simulink model "Robot_Control"  (R2023b)
settings: Solver=FixedStepDiscrete  StartTime=0.0  StopTime=inf  FixedStep=t_sample  RelTol=1e-3
undefined symbols (not defined in the file): t_sample
settings Model: Creator=FIRSTMentor  LastModifiedBy=ander
settings OptimizationCC: DefaultParameterBehavior=Inlined  StrengthReduction=on  PassReuseOutputArgsAs=Individual arguments  ZeroExternalMemoryAtStartup=off  ZeroInternalMemoryAtStartup=off  OptimizeBlockOrder=speed  OptimizationPriority=Speed  OptimizationCustomize=off  MultiThreadedLoops=on  EfficientTunableParamExpr=on
settings DebuggingCC: MergeDetectMultiDrivingBlocksExec=none  ParameterTunabilityLossMsg=error
settings HardwareCC: ProdBitPerPointer=32  ProdBitPerSizeT=32  ProdBitPerPtrDiffT=32  ProdLargestAtomicInteger=Long  ProdWordSize=32  ProdHWDeviceType=ARM Compatible->ARM 7
settings ModelReferenceCC: PropagateSignalLabelsOutOfModel=off
settings SFSimCC: MATLABDynamicMemAlloc=off
settings RTWCC: Description=Embedded Coder  SystemTargetFile=ert.tlc  GenCodeOnly=on  TemplateMakefile=ert_default_tmf  Toolchain=MinGW64 | gmake (64-bit Windows)
settings CodeAppCC: ForceParamTrailComments=on  IgnoreCustomStorageClasses=off  OperatorAnnotations=on  SimulinkDataObjDesc=on  SFDataObjDesc=on  InsertBlockDesc=on
settings ERTTargetCC: TargetLangStandard=C99 (ISO)  UtilityFuncGeneration=Shared location  SupportVariableSizeSignals=on  ParenthesesLevel=Maximum  InlinedParameterPlacement=NonHierarchical  ERTCustomFileTemplate=example_file_process.tlc

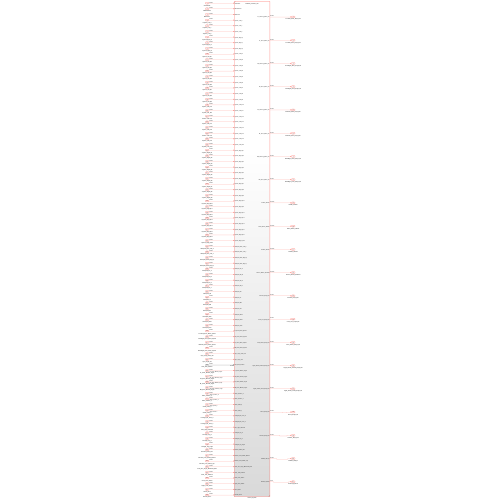
[thumbnail: Simulink's stored preview of the top-level diagram]
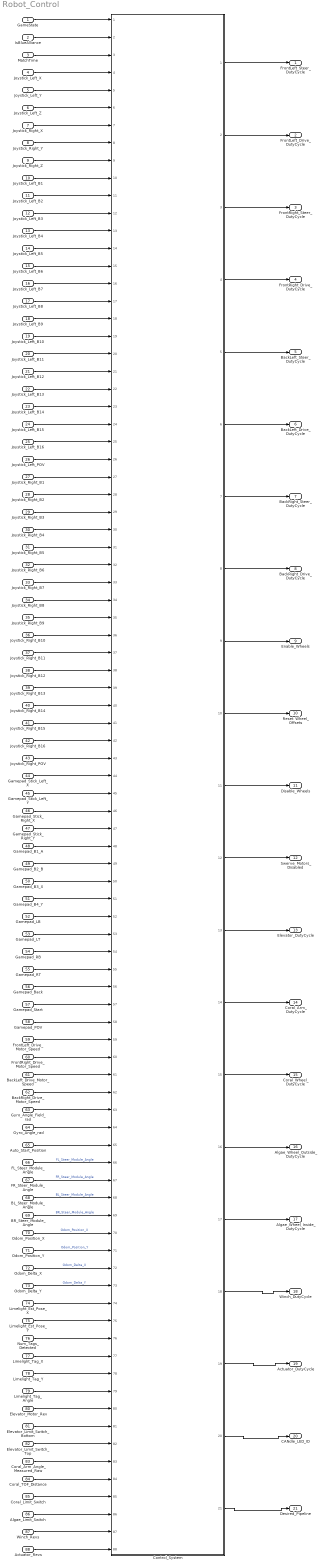
== system Robot_Control ==
  GameState : Inport
  IsBlueAlliance : Inport  Port=2
  MatchTime : Inport  Port=3
  Joystick_Left_X : Inport  Port=4
  Joystick_Left_Y : Inport  Port=5
  Joystick_Left_Z : Inport  Port=6
  Joystick_Right_X : Inport  Port=7
  Joystick_Right_Y : Inport  Port=8
  Joystick_Right_Z : Inport  Port=9
  Joystick_Left_B1 : Inport  Port=10
  Joystick_Left_B2 : Inport  Port=11
  Joystick_Left_B3 : Inport  Port=12
  Joystick_Left_B4 : Inport  Port=13
  Joystick_Left_B5 : Inport  Port=14
  Joystick_Left_B6 : Inport  Port=15
  Joystick_Left_B7 : Inport  Port=16
  Joystick_Left_B8 : Inport  Port=17
  Joystick_Left_B9 : Inport  Port=18
  Joystick_Left_B10 : Inport  Port=19
  Joystick_Left_B11 : Inport  Port=20
  Joystick_Left_B12 : Inport  Port=21
  Joystick_Left_B13 : Inport  Port=22
  Joystick_Left_B14 : Inport  Port=23
  Joystick_Left_B15 : Inport  Port=24
  Joystick_Left_B16 : Inport  Port=25
  Joystick_Left_POV : Inport  Port=26
  Joystick_Right_B1 : Inport  Port=27
  Joystick_Right_B2 : Inport  Port=28
  Joystick_Right_B3 : Inport  Port=29
  Joystick_Right_B4 : Inport  Port=30
  Joystick_Right_B5 : Inport  Port=31
  Joystick_Right_B6 : Inport  Port=32
  Joystick_Right_B7 : Inport  Port=33
  Joystick_Right_B8 : Inport  Port=34
  Joystick_Right_B9 : Inport  Port=35
  Joystick_Right_B10 : Inport  Port=36
  Joystick_Right_B11 : Inport  Port=37
  Joystick_Right_B12 : Inport  Port=38
  Joystick_Right_B13 : Inport  Port=39
  Joystick_Right_B14 : Inport  Port=40
  Joystick_Right_B15 : Inport  Port=41
  Joystick_Right_B16 : Inport  Port=42
  Joystick_Right_POV : Inport  Port=43
  Gamepad_Stick_Left_X : Inport  Port=44
  Gamepad_Stick_Left_Y : Inport  Port=45
  Gamepad_Stick_Right_X : Inport  Port=46
  Gamepad_Stick_Right_Y : Inport  Port=47
  Gamepad_B1_A : Inport  Port=48
  Gamepad_B2_B : Inport  Port=49
  Gamepad_B3_X : Inport  Port=50
  Gamepad_B4_Y : Inport  Port=51
  Gamepad_LB : Inport  Port=52
  Gamepad_LT : Inport  Port=53
  Gamepad_RB : Inport  Port=54
  Gamepad_RT : Inport  Port=55
  Gamepad_Back : Inport  Port=56
  Gamepad_Start : Inport  Port=57
  Gamepad_POV : Inport  Port=58
  FrontLeft_Drive_Motor_Speed : Inport  Port=59
  FrontRight_Drive_Motor_Speed : Inport  Port=60
  BackLeft_Drive_Motor_Speed : Inport  Port=61
  BackRight_Drive_Motor_Speed : Inport  Port=62
  Gyro_Angle_Field_rad : Inport  Port=63
  Gyro_Angle_rad : Inport  Port=64
  Auto_Start_Position : Inport  Port=65
  FL_Steer_Module_Angle : Inport  Port=66
  FR_Steer_Module_Angle : Inport  Port=67
  BL_Steer_Module_Angle : Inport  Port=68
  BR_Steer_Module_Angle : Inport  Port=69
  Odom_Position_X : Inport  Port=70
  Odom_Position_Y : Inport  Port=71
  Odom_Delta_X : Inport  Port=72
  Odom_Delta_Y : Inport  Port=73
  Limelight_Est_Pose_X : Inport  Port=74
  Limelight_Est_Pose_Y : Inport  Port=75
  Num_Tags_Detected : Inport  Port=76
  Limelight_Tag_X : Inport  Port=77
  Limelight_Tag_Y : Inport  Port=78
  Limelight_Tag_Angle : Inport  Port=79
  Elevator_Motor_Rev : Inport  Port=80
  Elevator_Limit_Switch_Bottom : Inport  Port=81
  Elevator_Limit_Switch_Top : Inport  Port=82
  Coral_Arm_Angle_Measured_Raw : Inport  Port=83
  Coral_TOF_Distance : Inport  Port=84
  Coral_Limit_Switch : Inport  Port=85
  Algae_Limit_Switch : Inport  Port=86
  Winch_Revs : Inport  Port=87
  Actuator_Revs : Inport  Port=88
  Control_System : Subsystem  SystemSampleTime=t_sample  RTWFcnName=Model_Step  ReferencedSubsystem=RoboRio_Controls_sub
      settings: RTWSystemCode=Nonreusable function  RTWFcnNameOpts=User specified
  FrontLeft_Steer_DutyCycle : Outport
  FrontLeft_Drive_DutyCycle : Outport  Port=2
  FrontRight_Steer_DutyCycle : Outport  Port=3
  FrontRight_Drive_DutyCycle : Outport  Port=4
  BackLeft_Steer_DutyCycle : Outport  Port=5
  BackLeft_Drive_DutyCycle : Outport  Port=6
  BackRight_Steer_DutyCycle : Outport  Port=7
  BackRight_Drive_DutyCycle : Outport  Port=8
  Enable_Wheels : Outport  Port=9
  Reset_Wheel_Offsets : Outport  Port=10
  Disable_Wheels : Outport  Port=11
  Swerve_Motors_Disabled : Outport  Port=12
  Elevator_DutyCycle : Outport  Port=13
  Coral_Arm_DutyCycle : Outport  Port=14
  Coral_Wheel_DutyCycle : Outport  Port=15
  Algae_Wheel_Outside_DutyCycle : Outport  Port=16
  Algae_Wheel_Inside_DutyCycle : Outport  Port=17
  Winch_DutyCycle : Outport  Port=18
  Actuator_DutyCycle : Outport  Port=19
  CANdle_LED_ID : Outport  Port=20
  Desired_Pipeline : Outport  Port=21
  wires:
  Odom_Delta_Y/1 -> Control_System/73  "Odom_Delta_Y"
  Joystick_Right_B5/1 -> Control_System/31
  Joystick_Left_POV/1 -> Control_System/26
  Joystick_Left_B16/1 -> Control_System/25
  Joystick_Left_B15/1 -> Control_System/24
  Joystick_Left_B13/1 -> Control_System/22
  Joystick_Left_B9/1 -> Control_System/18
  Joystick_Left_B11/1 -> Control_System/20
  Joystick_Left_B8/1 -> Control_System/17
  Joystick_Left_B7/1 -> Control_System/16
  Joystick_Left_B1/1 -> Control_System/10
  Joystick_Right_Z/1 -> Control_System/9
  Joystick_Right_Y/1 -> Control_System/8
  Joystick_Left_B3/1 -> Control_System/12
  Joystick_Left_Y/1 -> Control_System/5
  Joystick_Left_X/1 -> Control_System/4
  Joystick_Right_B7/1 -> Control_System/33
  Joystick_Right_B1/1 -> Control_System/27
  Joystick_Right_B2/1 -> Control_System/28
  Joystick_Right_B13/1 -> Control_System/39
  Joystick_Right_B8/1 -> Control_System/34
  Joystick_Right_B10/1 -> Control_System/36
  FrontRight_Drive_Motor_Speed/1 -> Control_System/60
  Control_System/14 -> Coral_Arm_DutyCycle/1
  MatchTime/1 -> Control_System/3
  Joystick_Left_B5/1 -> Control_System/14
  Joystick_Right_B4/1 -> Control_System/30
  Winch_Revs/1 -> Control_System/87
  Control_System/18 -> Winch_DutyCycle/1
  Control_System/6 -> BackLeft_Drive_DutyCycle/1
  Control_System/9 -> Enable_Wheels/1
  Elevator_Motor_Rev/1 -> Control_System/80
  Control_System/19 -> Actuator_DutyCycle/1
  Control_System/20 -> CANdle_LED_ID/1
  FrontLeft_Drive_Motor_Speed/1 -> Control_System/59
  Actuator_Revs/1 -> Control_System/88
  Gamepad_POV/1 -> Control_System/58
  Num_Tags_Detected/1 -> Control_System/76
  Limelight_Tag_Angle/1 -> Control_System/79
  Limelight_Tag_X/1 -> Control_System/77
  Gyro_Angle_Field_rad/1 -> Control_System/63
  Limelight_Tag_Y/1 -> Control_System/78
  Gamepad_Stick_Right_X/1 -> Control_System/46
  Elevator_Limit_Switch_Top/1 -> Control_System/82
  Gamepad_Start/1 -> Control_System/57
  Control_System/17 -> Algae_Wheel_Inside_DutyCycle/1
  Elevator_Limit_Switch_Bottom/1 -> Control_System/81
  Control_System/10 -> Reset_Wheel_Offsets/1
  Joystick_Right_B3/1 -> Control_System/29
  Gamepad_B2_B/1 -> Control_System/49
  Gamepad_RB/1 -> Control_System/54
  Coral_Arm_Angle_Measured_Raw/1 -> Control_System/83
  Control_System/1 -> FrontLeft_Steer_DutyCycle/1
  Control_System/4 -> FrontRight_Drive_DutyCycle/1
  Joystick_Left_B10/1 -> Control_System/19
  Joystick_Left_B12/1 -> Control_System/21
  Coral_Limit_Switch/1 -> Control_System/85
  IsBlueAlliance/1 -> Control_System/2
  Gamepad_RT/1 -> Control_System/55
  Joystick_Left_Z/1 -> Control_System/6
  Control_System/5 -> BackLeft_Steer_DutyCycle/1
  Control_System/21 -> Desired_Pipeline/1
  Joystick_Left_B14/1 -> Control_System/23
  Control_System/15 -> Coral_Wheel_DutyCycle/1
  Control_System/11 -> Disable_Wheels/1
  Control_System/16 -> Algae_Wheel_Outside_DutyCycle/1
  Control_System/7 -> BackRight_Steer_DutyCycle/1
  Joystick_Left_B4/1 -> Control_System/13
  Control_System/2 -> FrontLeft_Drive_DutyCycle/1
  BackRight_Drive_Motor_Speed/1 -> Control_System/62
  Joystick_Left_B6/1 -> Control_System/15
  Gamepad_Stick_Right_Y/1 -> Control_System/47
  Gamepad_B4_Y/1 -> Control_System/51
  Joystick_Right_B16/1 -> Control_System/42
  Gamepad_B1_A/1 -> Control_System/48
  Limelight_Est_Pose_Y/1 -> Control_System/75
  BackLeft_Drive_Motor_Speed/1 -> Control_System/61
  Coral_TOF_Distance/1 -> Control_System/84
  Gamepad_LT/1 -> Control_System/53
  Limelight_Est_Pose_X/1 -> Control_System/74
  Gamepad_B3_X/1 -> Control_System/50
  Joystick_Right_POV/1 -> Control_System/43
  Joystick_Right_B6/1 -> Control_System/32
  Joystick_Right_B15/1 -> Control_System/41
  Control_System/3 -> FrontRight_Steer_DutyCycle/1
  Joystick_Right_B14/1 -> Control_System/40
  Joystick_Right_B12/1 -> Control_System/38
  Control_System/13 -> Elevator_DutyCycle/1
  Joystick_Right_B11/1 -> Control_System/37
  Joystick_Right_B9/1 -> Control_System/35
  Control_System/12 -> Swerve_Motors_Disabled/1
  Algae_Limit_Switch/1 -> Control_System/86
  GameState/1 -> Control_System/1
  FL_Steer_Module_Angle/1 -> Control_System/66  "FL_Steer_Module_Angle"
  Odom_Delta_X/1 -> Control_System/72  "Odom_Delta_X"
  Gamepad_Stick_Left_Y/1 -> Control_System/45
  Gamepad_LB/1 -> Control_System/52
  Joystick_Left_B2/1 -> Control_System/11
  Gyro_Angle_rad/1 -> Control_System/64
  Odom_Position_Y/1 -> Control_System/71  "Odom_Position_Y"
  Odom_Position_X/1 -> Control_System/70  "Odom_Position_X"
  BR_Steer_Module_Angle/1 -> Control_System/69  "BR_Steer_Module_Angle"
  Gamepad_Stick_Left_X/1 -> Control_System/44
  BL_Steer_Module_Angle/1 -> Control_System/68  "BL_Steer_Module_Angle"
  Control_System/8 -> BackRight_Drive_DutyCycle/1
  Gamepad_Back/1 -> Control_System/56
  FR_Steer_Module_Angle/1 -> Control_System/67  "FR_Steer_Module_Angle"
  Joystick_Right_X/1 -> Control_System/7
  Auto_Start_Position/1 -> Control_System/65
